simulink model "test_DCM_block"  (R2018a)
settings: Solver=VariableStepAuto  StartTime=0.0  StopTime=10.0  RelTol=1e-3
libraries: simulink_extras x1, sharedtransform x1
settings Model: Creator=Jason  LastModifiedBy=Jason

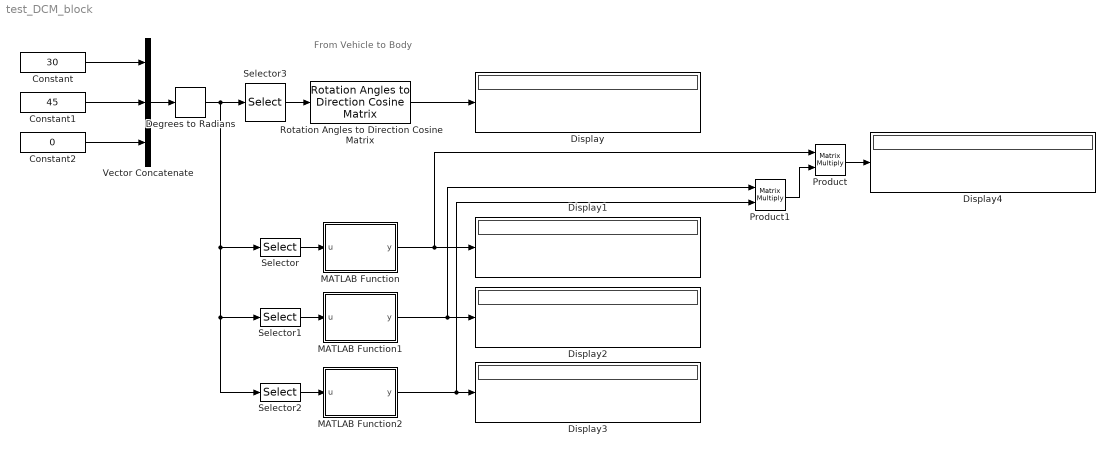
== system test_DCM_block ==
  note: From Vehicle to Body
  Constant : Constant  Value=30
  Constant1 : Constant  Value=45
  Constant2 : Constant  Value=0
  Degrees to Radians : simulink_extras/Transformations/Degrees to Radians
  Display{,1..4} (5 alike) : Display
  MATLAB Function : MATLAB Function  TreatAsAtomicUnit=on
  MATLAB Function1 : MATLAB Function  TreatAsAtomicUnit=on
  MATLAB Function2 : MATLAB Function  TreatAsAtomicUnit=on
  Product : Product  Multiplication=Matrix(*)
  Product1 : Product  Multiplication=Matrix(*)
  Rotation Angles to Direction Cosine Matrix : sharedtransform/Rotation Angles to Direction Cosine Matrix  rotationOrder=ZYX  aMode=aMode
      settings: SourceProductBaseCode=AE
  Selector : Selector  InputPortWidth=3  IndexOptions=Index vector (dialog)  Indices=1  OutputSizes=1
      settings: AttributesFormatString=|
      | %<IndexMode>
      | Index = %<Indices>
  Selector1 : Selector  InputPortWidth=3  IndexOptions=Index vector (dialog)  Indices=2  OutputSizes=1
      settings: AttributesFormatString=|
      | %<IndexMode>
      | Index = %<Indices>
  Selector2 : Selector  InputPortWidth=3  IndexOptions=Index vector (dialog)  Indices=3  OutputSizes=1
      settings: AttributesFormatString=|
      | %<IndexMode>
      | Index = %<Indices>
  Selector3 : Selector  InputPortWidth=3  IndexOptions=Index vector (dialog)  Indices=[3 2 1]  OutputSizes=1
  Vector Concatenate : Concatenate  NumInputs=3
  wires:
  Vector Concatenate/1 -> Degrees to Radians/1
  Degrees to Radians/1 -> Selector2/1, Selector1/1, Selector/1, Selector3/1
  Constant/1 -> Vector Concatenate/1
  Constant1/1 -> Vector Concatenate/2
  Constant2/1 -> Vector Concatenate/3
  Rotation Angles to Direction Cosine Matrix/1 -> Display/1
  Selector/1 -> MATLAB Function/1(u)
  Selector1/1 -> MATLAB Function1/1(u)
  Selector2/1 -> MATLAB Function2/1(u)
  MATLAB Function/1(y) -> Product/1, Display1/1
  MATLAB Function1/1(y) -> Product1/1, Display2/1
  MATLAB Function2/1(y) -> Product1/2, Display3/1
  Product1/1 -> Product/2
  Product/1 -> Display4/1
  Selector3/1 -> Rotation Angles to Direction Cosine Matrix/1

== matlab function test_DCM_block/MATLAB Function1 ==
  data: u input; y output
function y = fcn(u)

y = [
    cos(u) 0 -sin(u);
    0 1 0;
    sin(u) 0 cos(u);];

== matlab function test_DCM_block/MATLAB Function ==
  data: u input; y output
function y = fcn(u)

y = [
    1 0 0;
    0 cos(u) sin(u);
    0 -sin(u) cos(u);];

== matlab function test_DCM_block/MATLAB Function2 ==
  data: u input; y output
function y = fcn(u)


y = [
    cos(u) sin(u) 0;
    -sin(u) cos(u) 0;
    0 0 1;];
